simulink model "pendulum_pd"  (Simulink 6.3)
settings: Solver=ode45  StartTime=0.0  StopTime=10.0  RelTol=1e-3
settings Model: LastModifiedBy=Yuantao Gu

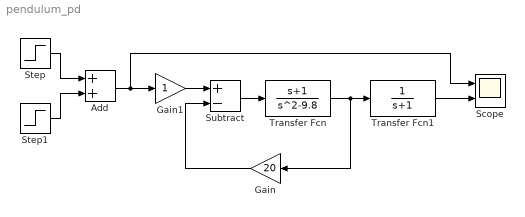
== system pendulum_pd ==
  Add : Sum  OutScaling=2^-10
  Gain : Gain  Orientation=left  Gain=20
  Gain1 : Gain
  Scope : Scope  NumInputPorts=2
      settings: YMin=-5~-5  YMax=5~5
  Step : Step  SampleTime=0
  Step1 : Step  Time=1.1  After=-1  SampleTime=0
  Subtract : Sum  Inputs=+-  OutScaling=2^-10
  Transfer Fcn : TransferFcn  Numerator=[1 1]  Denominator=[1 0 -9.8]
  Transfer Fcn1 : TransferFcn  Denominator=[1 1]
  wires:
  Gain1/1 -> Subtract/1
  Subtract/1 -> Transfer Fcn/1
  Transfer Fcn/1 -> Gain/1, Transfer Fcn1/1
  Gain/1 -> Subtract/2
  Step/1 -> Add/1
  Add/1 -> Gain1/1, Scope/1
  Step1/1 -> Add/2
  Transfer Fcn1/1 -> Scope/2
